simulink model "Reaching_Phantom"  (R2023b)
settings: Solver=FixedStepDiscrete  StartTime=0.0  StopTime=inf  FixedStep=0.001  RelTol=1e-3
libraries: PhanTorque_3Dof_Library_64Bits x1, vrlib x1
settings Model: Creator=carlos.aldana  LastModifiedBy=terri
settings SolverCC: AlgebraicLoopSolver=TrustRegion
settings DataIOCC: LimitDataPoints=on  SaveFormat=Array  ReturnWorkspaceOutputs=off
settings OptimizationCC: BlockReduction=off  BooleanDataType=off  LifeSpan=inf
settings DebuggingCC: SaveWithParameterizedLinksMsg=none  UnderspecifiedInitializationDetection=Classic  MergeDetectMultiDrivingBlocksExec=none  SignalResolutionControl=TryResolveAllWithWarning  UnconnectedInputMsg=warning  UnconnectedOutputMsg=warning  UnconnectedLineMsg=warning  AllowSymbolicDim=off  SFUnexpectedBacktrackingDiag=warning  SFNoUnconditionalDefaultTransitionDiag=warning  SFExecutionAtInitializationDiag=none  ArithmeticOperatorsInVariantConditions=warning
settings HardwareCC: ProdBitPerPointer=32  ProdBitPerSizeT=32  ProdBitPerPtrDiffT=32  ProdLargestAtomicFloat=None  ProdIntDivRoundTo=Undefined  ProdEndianess=Unspecified  ProdWordSize=32  ProdHWDeviceType=32-bit Generic  TargetUnknown=on
settings ModelReferenceCC: EnableRefExpFcnMdlSchedulingChecks=on  PropagateSignalLabelsOutOfModel=off
settings SFSimCC: SimUseLocalCustomCode=off  CustomCodeUndefinedFunction=UseInterfaceOnly
settings RTWCC: RTWUseLocalCustomCode=off  DLArmComputeVersion=19.05
settings CodeAppCC: StateflowObjectComments=on
settings GRTTargetCC: TargetLangStandard=C89/C90 (ANSI)
settings ConfigComp: CovMetricSettings=dw  CovSaveCumulativeToWorkspaceVar=on  CovSaveSingleToWorkspaceVar=on  CovExternalEMLEnable=off  CovSFcnEnable=off

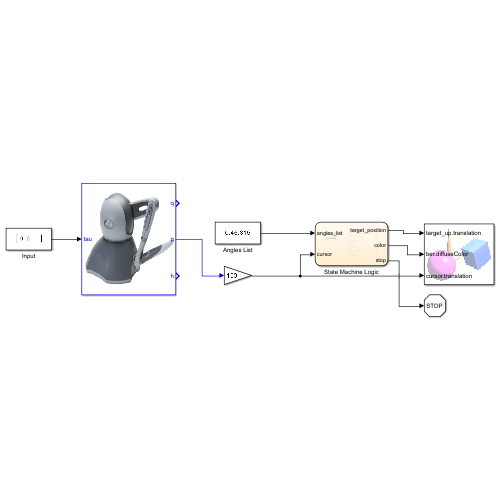
[thumbnail: Simulink's stored preview of the top-level diagram]
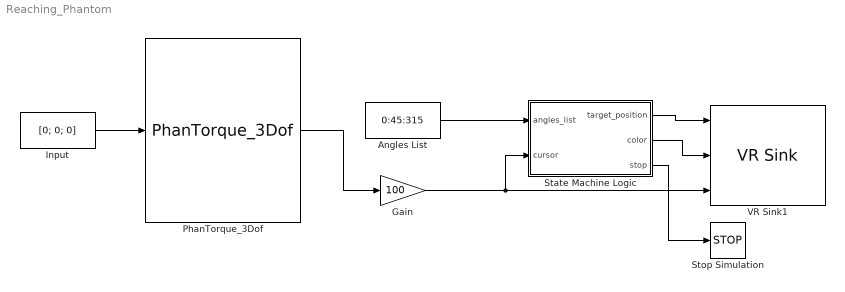
== system Reaching_Phantom ==
  Angles List : Constant  Value=0:45:315
  Gain : Gain  Gain=100
  Input : Constant  Value=[0; 0; 0]
  PhanTorque_3Dof : PhanTorque_3Dof_Library_64Bits/PhanTorque_3Dof  Haptic_Name='Default device'
  State Machine Logic : Stateflow chart  TreatAsAtomicUnit=on
      settings: PortSchema="{\"entries\":[{\"content\":{\"sides\":[{\"content\":{\"connectorIds\":[\"In1\",\"In2\"]},\"type\":\"ConnectorPlacement.EquallySpacedRectSide\",\"uuid\":\"2012c964-2602-4c80-977b-ac7ca7ae8f5b\"},{\"content\":{\"connectorIds\":[\"Out2\",\"Out1\",\"Out3\"],\"side\":\"RIGHT\"},\"type\":\"ConnectorPlacement.EquallySpacedRectSide\",\"uuid\":\"01c6fc3b-ba25-4dd7-b95f-3fc66d6fa31c\"},{\"content\":{\"side\":\"TOP\"},\"type\":\"ConnectorPlacement.EquallySpacedRectSide\",\"uuid\":\"0e349c8b-fff0-4cce-a38e-56f1937a9eb7\"}]},\"type\":\"ConnectorPlacement.EquallySpacedConnector\",\"uuid\":\"0aec7ed3-d29a-41fc-b2f0-597bb4555e1d\"}],\"packageUris\":[\"http://schema.mathworks.com/mf0/Connector/R2020b\"],\"version\":\"1.0\"}"
  Stop Simulation : Stop
  VR Sink1 : vrlib/VR Sink  InstantiateOnLoad=on  SampleTime=0.01  ViewEnable=on  RemoteChange=off  RemoteView=off  FieldsWritten=target_up.translation.3.1.1.double#ber.diffuseColor.3.1.1.double#cursor.translation.3.1.1.double  WorldFileName=2_palline_color.wrl  AutoView=off  VideoDimensions=[]  AllowVariableSize=off  FigureProperties=[]
  wires:
  Input/1 -> PhanTorque_3Dof/1
  PhanTorque_3Dof/2 -> Gain/1
  State Machine Logic/3(stop) -> Stop Simulation/1
  Angles List/1 -> State Machine Logic/1(angles_list)
  Gain/1 -> State Machine Logic/2(cursor), VR Sink1/3
  State Machine Logic/2(target_position) -> VR Sink1/1
  State Machine Logic/1(color) -> VR Sink1/2

== stateflow chart Reaching_Phantom/State Machine Logic ==
  state Start
    entry:
    index = 1;
  state RandomAngleGeneration
    entry:
    random_angles_list = randomAngle(angles_list);
    idx = 1;
  state ShowTarget
    entry:
    color = [1 0.2 0.2];
    target_position = computeTargetPose(random_angles_list(idx));
  state ChangeToReachingColor
    entry:
    color = [0 0.8 1];
  state ReturnToStartPosition
    entry:
    target_position = [0 0 0];
    color = [1 0.2 0.2];
  state ChangeToReachingColor2
    entry:
    color = [0 0.8 1];
  state Finish
    stop = 1;
  (default) -> Start [order 1]
  (default) -> Start [order 2]
  Start -> RandomAngleGeneration
  (junction 73) -> RandomAngleGeneration
  (junction 72) -> (junction 73)
  RandomAngleGeneration -> ShowTarget
  (junction 78) -> ShowTarget : after(2, sec)[sqrt((target_position(1)-cursor(1))^2 + (target_position(2)-cursor(2))^2) <= 0.2 & i < 2 & idx ~= 8]{idx = idx + 1}
  ShowTarget -> ChangeToReachingColor : [sqrt((target_position(1)-cursor(1))^2 + (target_position(2)-cursor(2))^2) <= 0.2 & idx <= 8]
  ChangeToReachingColor -> ShowTarget [order 1] : [sqrt((target_position(1)-cursor(1))^2 + (target_position(2)-cursor(2))^2) > 0.2 ]
  ChangeToReachingColor -> ReturnToStartPosition [order 2] : after(2, sec)[sqrt((target_position(1)-cursor(1))^2 + (target_position(2)-cursor(2))^2) <= 0.2]
  ReturnToStartPosition -> ChangeToReachingColor2 : [sqrt((target_position(1)-cursor(1))^2 + (target_position(2)-cursor(2))^2) <= 0.2]
  ChangeToReachingColor2 -> ReturnToStartPosition [order 1] : [sqrt((target_position(1)-cursor(1))^2 + (target_position(2)-cursor(2))^2) > 0.2]
  ChangeToReachingColor2 -> (junction 78) [order 4]
  ChangeToReachingColor2 -> Finish [order 2] : [idx == 2 & index == 2]
  ChangeToReachingColor2 -> (junction 76) [order 3]
  (junction 76) -> (junction 72) : after(2, sec)[idx == 8 & sqrt((target_position(1)-cursor(1))^2 + (target_position(2)-cursor(2))^2) < 0.2 ]{index = index+1}
  data: al function_input; random_list function_output; angle function_input; r function_output; angles_list input; color output; cursor input; target_position output; idx local; random_angles_list local; index local; stop output =0
  function random_list = randomAngle(al):
    | function random_list = randomAngle(al)
    |     size_list = length(al);
    |     random_index = randperm(size_list);
    |     
    |     % Inizializza la nuova lista con le stesse dimensioni di al
    |     new_list = zeros(size_list, 1);
    | 
    |     for i = 1:size_list
    |         % Assegna gli elementi di al nell'ordine casuale
    |         new_list(i) = al(random_index(i));
    |     end
    | 
    |     random_list = new_list;
    | end
  function r = computeTargetPose(angle):
    | function r = computeTargetPose(angle)
    |     % Converti l'angolo da gradi a radianti
    |     theta = deg2rad(angle);
    | 
    |     % Calcola le coordinate del punto sulla circonferenza
    |     x = 10 * cos(theta);
    |     y = 10 * sin(theta);
    |     z = 0;
    |     r =[x y z];
    | end
